simulink model "Single_Phase_SAPF_10mar2018_HCC"  (R2017a)
settings: Solver=ode45  StartTime=0.0  StopTime=5  RelTol=1e-3  EnableMultiTasking=on
undefined symbols (not defined in the file or in its folder): DiscIntNeverNeededParam
libraries: powerlib x21, powerlib_meascontrol x2
settings Model: Creator=Niranjan  LastModifiedBy=Dell
settings DataIOCC: LimitDataPoints=on  SaveFormat=Array
settings OptimizationCC: LifeSpan=inf
settings DebuggingCC: SolverPrmCheckMsg=warning  SFUnexpectedBacktrackingDiag=warning  SFNoUnconditionalDefaultTransitionDiag=warning  SFExecutionAtInitializationDiag=none
settings HardwareCC: ProdBitPerPointer=32  ProdBitPerSizeT=32  ProdBitPerPtrDiffT=32  ProdLargestAtomicFloat=None  ProdIntDivRoundTo=Undefined  ProdEndianess=Unspecified  ProdWordSize=32  ProdHWDeviceType=32-bit Generic
settings ModelReferenceCC: PropagateSignalLabelsOutOfModel=off
settings GRTTargetCC: TargetLangStandard=C89/C90 (ANSI)  GeneratePreprocessorConditionals=Disable all
settings ConfigComp: CovMetricSettings=dw  CovHtmlReporting=on  CovSaveCumulativeToWorkspaceVar=on  CovSaveSingleToWorkspaceVar=on  CovExternalEMLEnable=off  CovSFcnEnable=off

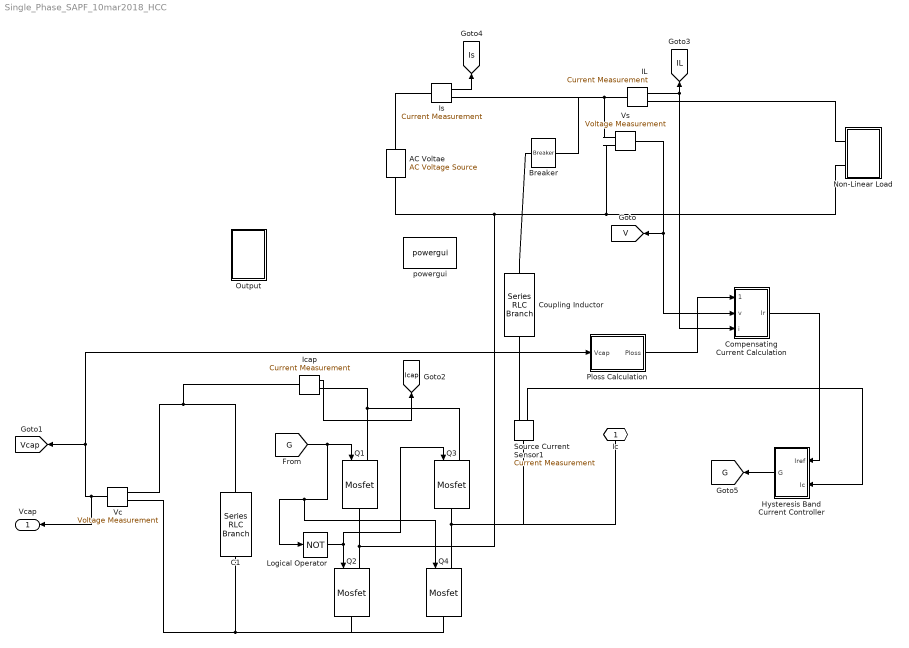
== system Single_Phase_SAPF_10mar2018_HCC ==
  AC Voltae : powerlib/Electrical Sources/AC Voltage Source  Amplitude=311  Phase=0  Frequency=50  SampleTime=0  Measurements=None  BusType=swing  Pref=10e3  Qref=0  Qmin=-inf  Qmax=+inf
  Breaker : powerlib/Elements/Breaker  InitialState=0  SwitchingTimes=[1]  External=off  BreakerResistance=0.001  SnubberResistance=1e7  SnubberCapacitance=inf  Measurements=None  MoreParameters=on  NoBreakLoop=off
      settings: SourceProductName=Simscape Power Systems
  C1 : powerlib/Elements/Series RLC Branch  LConnTagsString=__new0  RConnTagsString=__new0  BranchType=C  Resistance=1  Inductance=0.04  SetiL0=off  InitialCurrent=0  Capacitance=10000e-6  Setx0=on  InitialVoltage=400  Measurements=None
  Compensating Current Calculation : Subsystem
  Coupling Inductor : powerlib/Elements/Series RLC Branch  LConnTagsString=__new0  RConnTagsString=__new0  BranchType=L  Resistance=0.01  Inductance=0.5e-3  SetiL0=off  InitialCurrent=0  Capacitance=0.015  Setx0=off  InitialVoltage=0  Measurements=None
  Hysteresis Band Current Controller : Subsystem
  IL : powerlib/Measurements/Current Measurement  PhasorSimulation=off  OutputType=Complex  PSBequivalent=0
  Icap : powerlib/Measurements/Current Measurement  PhasorSimulation=off  OutputType=Complex  PSBequivalent=0
  Is : powerlib/Measurements/Current Measurement  PhasorSimulation=off  OutputType=Complex  PSBequivalent=0
  Logical Operator : Logic  Operator=NOT  AllPortsSameDT=off  OutDataTypeStr=boolean
  Non-Linear Load : Subsystem
  Output : Subsystem
  Ploss Calculation : Subsystem
  Q{1..4} (4 alike) : powerlib/Power Electronics/Mosfet  Ron=0.1  Lon=0  Rd=0.01  Vfd=0  IC=0  Rs=1e5  Cs=inf  Measurements=off
  Source Current Sensor1 : powerlib/Measurements/Current Measurement  PhasorSimulation=off  OutputType=Complex  PSBequivalent=0
  Vc : powerlib/Measurements/Voltage Measurement  PhasorSimulation=off  OutputType=Complex  PSBequivalent=0
  Vs : powerlib/Measurements/Voltage Measurement  PhasorSimulation=off  OutputType=Complex  PSBequivalent=0
  powergui : powerlib/powergui  Priority=1  SimulationMode=Discrete  SampleTime=1e-6  frequency=60  Iterations=50  frequencyindice=50  Pbase=100e6  ErrMax=1e-4  UnitsV=kV  UnitsW=MW  buscounter=0  FunctionMessages=off  echomessages=off  EnableUseOfTLC=off  CurrentSourceSwitches=off  DisableSnubberDevices=off  DisableRonSwitches=off  DisableVfSwitches=off  DisplayEquations=off  SolverType=Tustin/Backward Euler (TBE)  Interpol=off  ExternalGateDelay=off  methode=off  Ts=10  x0status=blocks  SPID=off  SwTol=0  HookPort=off  RestoreLinks=warning  ResistiveCurrentMeasurement=off  Frange=[0:2:500]  Ylog=off  Xlog=on  ShowGrid=off  save=off  variable=ZData  structure=0  ZoomFFT=off  StartTime=0.0  cycles=1  DisplayStyle=1  fundamental=60  FreqAxis=off  MaxFrequency=1000  frequencyindicesteady=1  RmsSteady=1  display=off
  Ic : PMIOPort  Port=1  Side=Right
  Vcap : Outport
  tag scope: G=global, IL=global, Icap=global, Is=global, V=global, Vcap=global
  wires:
  IL/1 -> Compensating Current Calculation/3(i), [IL]
  Vs/1 -> Compensating Current Calculation/2(v), [V]
  Is/1 -> [Is]
  Source Current Sensor1/1 -> Hysteresis Band Current Controller/2(Ic)
  Vc/1 -> Vcap/1, Ploss Calculation/1(Vcap), [Vcap]
  Ploss Calculation/1(Ploss) -> Compensating Current Calculation/1(Ploss)
  Compensating Current Calculation/1(Ir) -> Hysteresis Band Current Controller/1(Iref)
  Logical Operator/1 -> Q3/1, Q2/1
  Icap/1 -> [Icap]
  Hysteresis Band Current Controller/1(G) -> [G]
  [G] -> Q4/1, Logical Operator/1, Q1/1
  connections:
  IL/LConn1 -- Breaker/RConn1 -- Is/RConn1 -- Vs/LConn1
  Is/LConn1 -- AC Voltae/RConn1
  Source Current Sensor1/RConn1 -- Coupling Inductor/RConn1
  Non-Linear Load/LConn1 -- IL/RConn1
  Icap/RConn1 -- Q1/LConn1 -- Q3/LConn1
  Vc/LConn2 -- Q4/RConn1 -- Q2/RConn1 -- C1/RConn1
  Q3/RConn1 -- Source Current Sensor1/LConn1 -- Ic/RConn1 -- Q4/LConn1
  C1/LConn1 -- Icap/LConn1 -- Vc/LConn1
  AC Voltae/LConn1 -- Non-Linear Load/LConn2 -- Vs/LConn2 -- Q2/LConn1 -- Q1/RConn1
  Coupling Inductor/LConn1 -- Breaker/LConn1

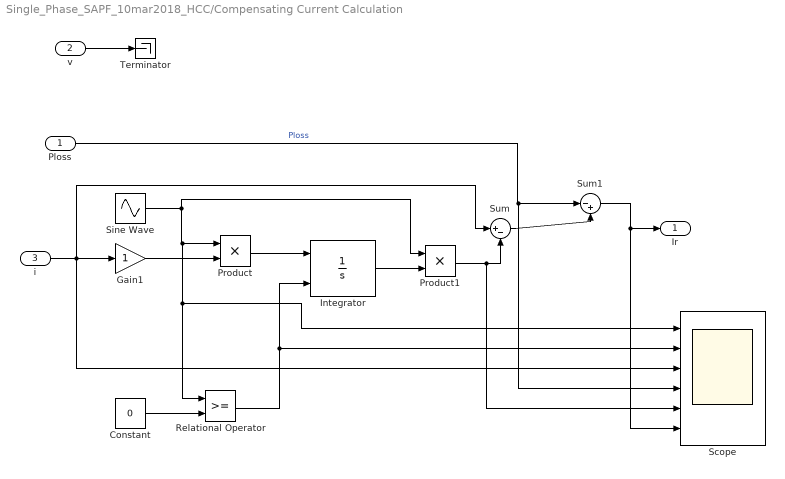
== system Single_Phase_SAPF_10mar2018_HCC/Compensating Current Calculation ==
  Ploss : Inport
  v : Inport  Port=2
  i : Inport  Port=3
  Constant : Constant  Value=0
  Gain1 : Gain
  Integrator : Integrator  ExternalReset=either
  Product : Product
  Product1 : Product
  Relational Operator : RelationalOperator  OutDataTypeStr=boolean  RndMeth=Simplest
  Scope : Scope  NumInputPorts=6
  Sine Wave : Sin  Frequency=314.16  SampleTime=0
  Sum : Sum  Inputs=|+-
  Sum1 : Sum  Inputs=|-+
  Terminator : Terminator
  Ir : Outport
  wires:
  i/1 -> Scope/3, Sum/1, Gain1/1
  Gain1/1 -> Product/2
  Sine Wave/1 -> Product/1, Relational Operator/1, Scope/1, Product1/1
  Product/1 -> Integrator/1
  Integrator/1 -> Product1/2
  v/1 -> Terminator/1
  Product1/1 -> Scope/5, Sum/2
  Sum/1 -> Sum1/2
  Ploss/1 -> Scope/4, Sum1/1  "Ploss"
  Sum1/1 -> Scope/6, Ir/1
  Relational Operator/1 -> Integrator/2, Scope/2
  Constant/1 -> Relational Operator/2

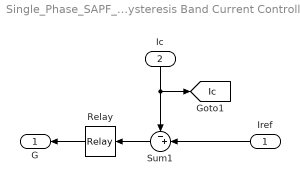
== system Single_Phase_SAPF_10mar2018_HCC/Hysteresis Band Current Controller ==
  Iref : Inport
  Ic : Inport  Port=2
  Relay : Relay  OnSwitchValue=0.1  OffSwitchValue=-0.1  ZeroCross=off
  Sum1 : Sum  Inputs=-+|
  G : Outport
  tag scope: Ic=global
  wires:
  Relay/1 -> G/1
  Ic/1 -> Sum1/1, [Ic]
  Sum1/1 -> Relay/1
  Iref/1 -> Sum1/2

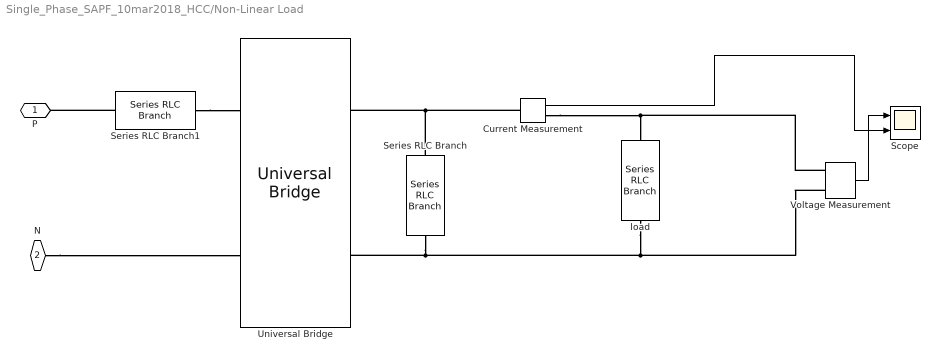
== system Single_Phase_SAPF_10mar2018_HCC/Non-Linear Load ==
  " load" : powerlib/Elements/Series RLC Branch  LConnTagsString=__new0  RConnTagsString=__new0  BranchType=R  Resistance=100  Inductance=1e-3  SetiL0=off  InitialCurrent=0  Capacitance=0.015  Setx0=off  InitialVoltage=0  Measurements=None
  Current Measurement : powerlib/Measurements/Current Measurement  PhasorSimulation=off  OutputType=Complex  PSBequivalent=0
  Scope : Scope  NumInputPorts=2
  Series RLC Branch : powerlib/Elements/Series RLC Branch  LConnTagsString=__new0  RConnTagsString=__new0  BranchType=C  Resistance=1  Inductance=1e-3  SetiL0=off  InitialCurrent=0  Capacitance=3300e-6  Setx0=on  InitialVoltage=235  Measurements=None
  Series RLC Branch1 : powerlib/Elements/Series RLC Branch  LConnTagsString=__new0  RConnTagsString=__new0  BranchType=L  Resistance=1  Inductance=1e-3  SetiL0=off  InitialCurrent=4  Capacitance=1e-6  Setx0=off  InitialVoltage=0  Measurements=None
  Universal Bridge : powerlib/Power Electronics/Universal Bridge  Arms=2  SnubberResistance=1e5  SnubberCapacitance=inf  Device=Diodes  Ron=1e-3  Lon=0  ForwardVoltages="[  0  0  ]"  ForwardVoltage=0  GTOparameters=[ 10e-6 , 20e-6 ]  IGBTparameters=[ 1e-6 , 2e-6 ]  Measurements=None  Measurements_2=None  converterType=Rectifier
  Voltage Measurement : powerlib/Measurements/Voltage Measurement  PhasorSimulation=off  OutputType=Complex  PSBequivalent=0
  P : PMIOPort  Port=1  Side=Left
  N : PMIOPort  Port=2  Side=Left
  wires:
  Voltage Measurement/1 -> Scope/1
  Current Measurement/1 -> Scope/2
  connections:
  Current Measurement/RConn1 -- Voltage Measurement/LConn1 -- " load"/LConn1
  Universal Bridge/RConn2 -- Voltage Measurement/LConn2 -- " load"/RConn1 -- Series RLC Branch/RConn1
  Current Measurement/LConn1 -- Series RLC Branch/LConn1 -- Universal Bridge/RConn1
  N/RConn1 -- Universal Bridge/LConn2
  Series RLC Branch1/RConn1 -- Universal Bridge/LConn1
  Series RLC Branch1/LConn1 -- P/RConn1

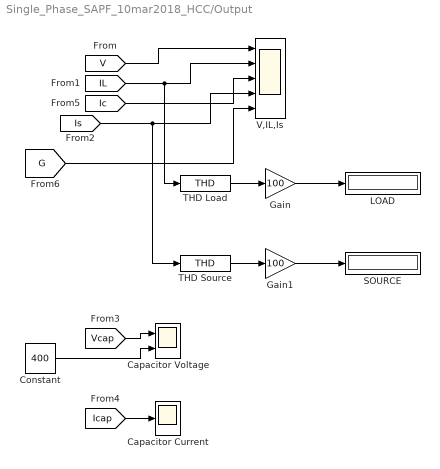
== system Single_Phase_SAPF_10mar2018_HCC/Output ==
  Capacitor Current : Scope
  Capacitor Voltage : Scope  NumInputPorts=2
  Constant : Constant  Value=400
  Gain : Gain  Gain=100
  Gain1 : Gain  Gain=100
  LOAD : Display
  SOURCE : Display
  THD Load : powerlib_meascontrol/Measurements/THD  Freq=50  Ts=0
  THD Source : powerlib_meascontrol/Measurements/THD  Freq=50  Ts=0
  V,IL,Is : Scope  NumInputPorts=5
  wires:
  [V] -> V,IL,Is/1
  [Vcap] -> Capacitor Voltage/1
  [Icap] -> Capacitor Current/1
  [Ic] -> V,IL,Is/3
  [Is] -> THD Source/1, V,IL,Is/4
  [IL] -> THD Load/1, V,IL,Is/2
  Gain/1 -> LOAD/1
  Gain1/1 -> SOURCE/1
  THD Load/1 -> Gain/1
  THD Source/1 -> Gain1/1
  Constant/1 -> Capacitor Voltage/2
  [G] -> V,IL,Is/5

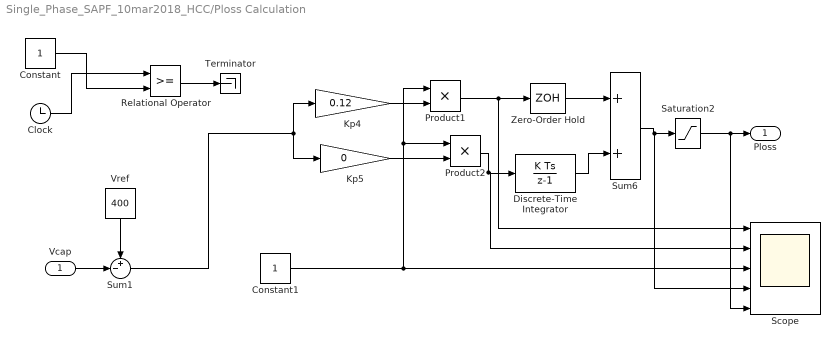
== system Single_Phase_SAPF_10mar2018_HCC/Ploss Calculation ==
  Vcap : Inport
  Clock : Clock
  Constant : Constant
  Constant1 : Constant
  Discrete-Time Integrator : DiscreteIntegrator  SampleTime=1e-6  LimitOutput=on  UpperSaturationLimit=1e6  LowerSaturationLimit=-1e6  ICPrevOutput=DiscIntNeverNeededParam  ICPrevScaledInput=DiscIntNeverNeededParam
  Kp4 : Gain  Gain=0.12  SaturateOnIntegerOverflow=on  OutDataTypeStr=Inherit: Same as input  ParamDataTypeStr=Inherit: Same as input
  Kp5 : Gain  Gain=0  SaturateOnIntegerOverflow=on  OutDataTypeStr=Inherit: Same as input  ParamDataTypeStr=Inherit: Same as input
  Product1 : Product
  Product2 : Product
  Relational Operator : RelationalOperator  OutDataTypeStr=boolean  RndMeth=Simplest
  Saturation2 : Saturate  UpperLimit=1e10  LowerLimit=-1e10
  Scope : Scope  NumInputPorts=5
  Sum1 : Sum  Inputs=+-|
  Sum6 : Sum  SaturateOnIntegerOverflow=on  InputSameDT=on  OutDataTypeStr=Inherit: Same as first input
  Terminator : Terminator
  Vref : Constant  Value=400
  Zero-Order Hold : ZeroOrderHold  SampleTime=1e-6
  Ploss : Outport
  wires:
  Vref/1 -> Sum1/1
  Vcap/1 -> Sum1/2
  Saturation2/1 -> Scope/5, Ploss/1
  Relational Operator/1 -> Terminator/1
  Clock/1 -> Relational Operator/1
  Constant/1 -> Relational Operator/2
  Sum6/1 -> Scope/4, Saturation2/1
  Zero-Order Hold/1 -> Sum6/1
  Discrete-Time Integrator/1 -> Sum6/2
  Sum1/1 -> Kp5/1, Kp4/1
  Kp5/1 -> Product2/2
  Kp4/1 -> Product1/2
  Product1/1 -> Scope/1, Zero-Order Hold/1
  Constant1/1 -> Scope/3, Product2/1, Product1/1
  Product2/1 -> Scope/2, Discrete-Time Integrator/1
